simulink model "Task2"  (R2016a)
settings: Solver=VariableStepAuto  StartTime=0.0  StopTime=10.0  RelTol=1e-3
settings Model: Creator=Thomas  LastModifiedBy=Thomas

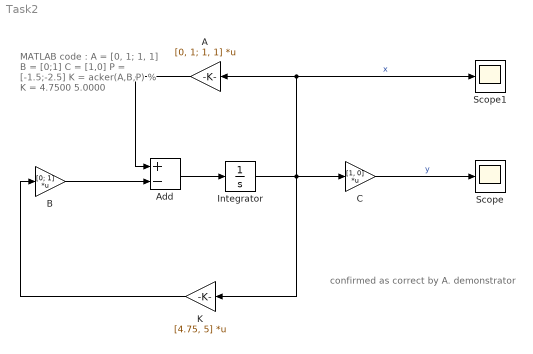
== system Task2 ==
  note: MATLAB code :
      | A = [0, 1; 1, 1]
      | B = [0;1]
      | C = [1,0]
      | P = [-1.5;-2.5]
      | K = acker(A,B,P)
      | % K = 4.7500 5.0000
  note: confirmed as correct by A. demonstrator
  A : Gain  Gain=[0, 1; 1, 1]  Multiplication=Matrix(K*u)
  Add : Sum  Inputs=+-
  B : Gain  Gain=[0; 1]  Multiplication=Matrix(K*u)
  C : Gain  Gain=[1, 0]  Multiplication=Matrix(K*u)
  Integrator : Integrator  InitialCondition=[1;1]
  K : Gain  Gain=[4.75, 5]  Multiplication=Matrix(K*u)
  Scope : Scope
  Scope1 : Scope
  wires:
  Add/1 -> Integrator/1
  A/1 -> Add/1
  B/1 -> Add/2
  Integrator/1 -> K/1, A/1, Scope1/1, C/1  "x"
  C/1 -> Scope/1  "y"
  K/1 -> B/1
